simulink model "CMM_iCub_23_25_DoFs"  (Simulink 9.0)
settings: Solver=VariableStepAuto  StartTime=0.0  StopTime=10.0  RelTol=1e-3
libraries: WBToolboxLibrary x31
settings Model: SuppressorTable=22 serialization::archive 11 0 6 0 0 0 1 0  Creator=gnava  LastModifiedBy=gnava
settings DataIOCC: SaveFormat=Dataset
settings OptimizationCC: LifeSpan=auto
settings DebuggingCC: UnderspecifiedInitializationDetection=Simplified  MergeDetectMultiDrivingBlocksExec=error  SFUnexpectedBacktrackingDiag=error  SFNoUnconditionalDefaultTransitionDiag=error  SFExecutionAtInitializationDiag=warning
settings HardwareCC: ProdBitPerPointer=64  ProdBitPerSizeT=64  ProdBitPerPtrDiffT=64  ProdLargestAtomicFloat=Float  ProdIntDivRoundTo=Zero  ProdEndianess=LittleEndian  ProdWordSize=64  ProdHWDeviceType=Intel->x86-64 (Windows64)
settings ModelReferenceCC: PropagateSignalLabelsOutOfModel=on
settings CodeAppCC: StateflowObjectComments=off
settings GRTTargetCC: TargetLangStandard=C99 (ISO)
settings ConfigComp: CovMetricSettings=dwe  CovHtmlReporting=off  CovSaveCumulativeToWorkspaceVar=off  CovSaveSingleToWorkspaceVar=off  CovExternalEMLEnable=on

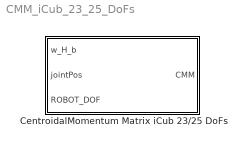
== system CMM_iCub_23_25_DoFs ==
  CentroidalMomentum Matrix iCub 23/25 DoFs : Subsystem

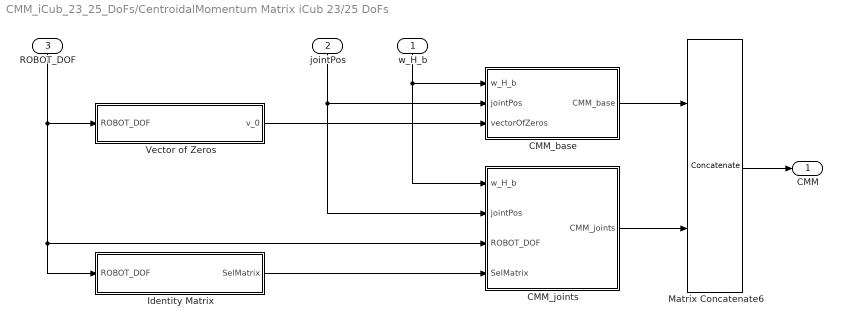
== system CMM_iCub_23_25_DoFs/CentroidalMomentum Matrix iCub 23/25 DoFs ==
  w_H_b : Inport
  jointPos : Inport  Port=2
  ROBOT_DOF : Inport  Port=3
  CMM_base : Subsystem
  CMM_joints : Subsystem
  Identity Matrix : MATLAB Function  TreatAsAtomicUnit=on
  Matrix Concatenate6 : Concatenate  Mode=Multidimensional array  ConcatenateDimension=2
  Vector of Zeros : MATLAB Function  TreatAsAtomicUnit=on
  CMM : Outport
  wires:
  Matrix Concatenate6/1 -> CMM/1
  CMM_base/1(CMM_base) -> Matrix Concatenate6/1
  jointPos/1 -> CMM_joints/2(jointPos), CMM_base/2(jointPos)
  w_H_b/1 -> CMM_joints/1(w_H_b), CMM_base/1(w_H_b)
  ROBOT_DOF/1 -> CMM_joints/3(ROBOT_DOF), Identity Matrix/1(ROBOT_DOF), Vector of Zeros/1(ROBOT_DOF)
  Vector of Zeros/1(v_0) -> CMM_base/3(vectorOfZeros)
  CMM_joints/1(CMM_joints) -> Matrix Concatenate6/2
  Identity Matrix/1(SelMatrix) -> CMM_joints/4(SelMatrix)

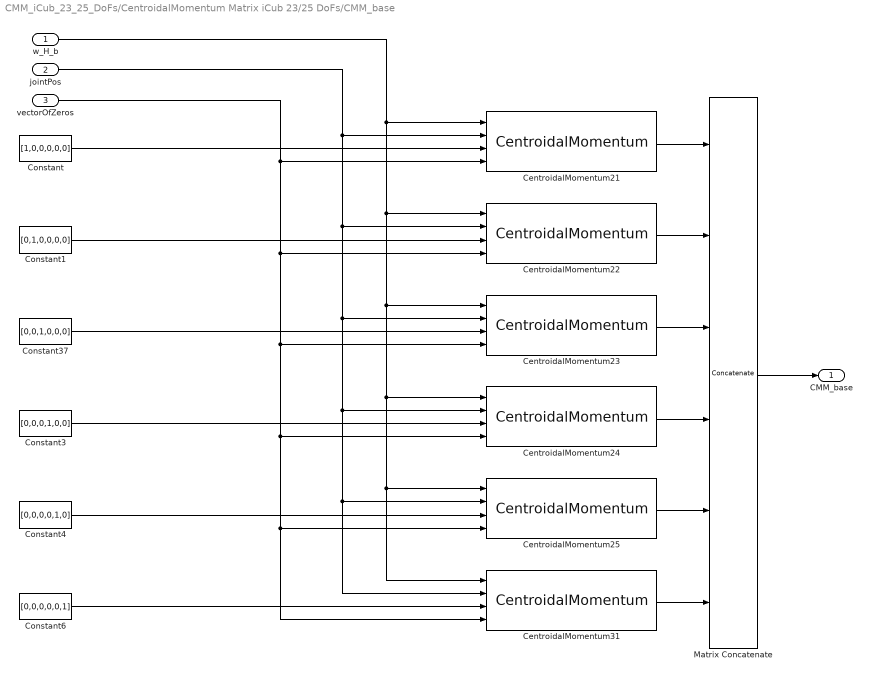
== system CMM_iCub_23_25_DoFs/CentroidalMomentum Matrix iCub 23/25 DoFs/CMM_base ==
  w_H_b : Inport
  jointPos : Inport  Port=2
  vectorOfZeros : Inport  Port=3
  CentroidalMomentum{21..25,31} (6 alike) : WBToolboxLibrary/Model/Dynamics/CentroidalMomentum
      settings: SourceProductName=WholeBodyToolbox
  Constant : Constant  Value=[1,0,0,0,0,0]
  Constant1 : Constant  Value=[0,1,0,0,0,0]
  Constant3 : Constant  Value=[0,0,0,1,0,0]
  Constant37 : Constant  Value=[0,0,1,0,0,0]
  Constant4 : Constant  Value=[0,0,0,0,1,0]
  Constant6 : Constant  Value=[0,0,0,0,0,1]
  Matrix Concatenate : Concatenate  NumInputs=6  Mode=Multidimensional array  ConcatenateDimension=2
  CMM_base : Outport
  wires:
  w_H_b/1 -> CentroidalMomentum31/1, CentroidalMomentum25/1, CentroidalMomentum24/1, CentroidalMomentum23/1, CentroidalMomentum22/1, CentroidalMomentum21/1
  jointPos/1 -> CentroidalMomentum31/2, CentroidalMomentum25/2, CentroidalMomentum24/2, CentroidalMomentum23/2, CentroidalMomentum22/2, CentroidalMomentum21/2
  CentroidalMomentum25/1 -> Matrix Concatenate/5
  Matrix Concatenate/1 -> CMM_base/1
  CentroidalMomentum23/1 -> Matrix Concatenate/3
  CentroidalMomentum24/1 -> Matrix Concatenate/4
  CentroidalMomentum31/1 -> Matrix Concatenate/6
  Constant6/1 -> CentroidalMomentum31/3
  Constant/1 -> CentroidalMomentum21/3
  Constant1/1 -> CentroidalMomentum22/3
  Constant37/1 -> CentroidalMomentum23/3
  vectorOfZeros/1 -> CentroidalMomentum21/4, CentroidalMomentum31/4, CentroidalMomentum25/4, CentroidalMomentum24/4, CentroidalMomentum23/4, CentroidalMomentum22/4
  Constant4/1 -> CentroidalMomentum25/3
  Constant3/1 -> CentroidalMomentum24/3
  CentroidalMomentum22/1 -> Matrix Concatenate/2
  CentroidalMomentum21/1 -> Matrix Concatenate/1

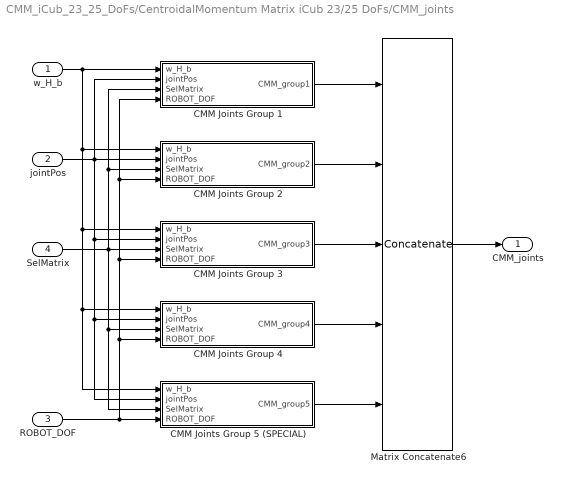
== system CMM_iCub_23_25_DoFs/CentroidalMomentum Matrix iCub 23/25 DoFs/CMM_joints ==
  w_H_b : Inport
  jointPos : Inport  Port=2
  ROBOT_DOF : Inport  Port=3
  SelMatrix : Inport  Port=4
  CMM Joints Group 1 : Subsystem
  CMM Joints Group 2 : Subsystem
  CMM Joints Group 3 : Subsystem
  CMM Joints Group 4 : Subsystem
  CMM Joints Group 5 (SPECIAL) : Subsystem
  Matrix Concatenate6 : Concatenate  NumInputs=5  Mode=Multidimensional array  ConcatenateDimension=2
  CMM_joints : Outport
  wires:
  Matrix Concatenate6/1 -> CMM_joints/1
  w_H_b/1 -> CMM Joints Group 1/1(w_H_b), CMM Joints Group 2/1(w_H_b), CMM Joints Group 3/1(w_H_b), CMM Joints Group 4/1(w_H_b), CMM Joints Group 5 (SPECIAL)/1(w_H_b)
  jointPos/1 -> CMM Joints Group 3/2(jointPos), CMM Joints Group 4/2(jointPos), CMM Joints Group 5 (SPECIAL)/2(jointPos), CMM Joints Group 2/2(jointPos), CMM Joints Group 1/2(jointPos)
  SelMatrix/1 -> CMM Joints Group 4/3(SelMatrix), CMM Joints Group 5 (SPECIAL)/3(SelMatrix), CMM Joints Group 3/3(SelMatrix), CMM Joints Group 2/3(SelMatrix), CMM Joints Group 1/3(SelMatrix)
  CMM Joints Group 1/1(CMM_group1) -> Matrix Concatenate6/1
  CMM Joints Group 2/1(CMM_group2) -> Matrix Concatenate6/2
  CMM Joints Group 3/1(CMM_group3) -> Matrix Concatenate6/3
  CMM Joints Group 4/1(CMM_group4) -> Matrix Concatenate6/4
  CMM Joints Group 5 (SPECIAL)/1(CMM_group5) -> Matrix Concatenate6/5
  ROBOT_DOF/1 -> CMM Joints Group 5 (SPECIAL)/4(ROBOT_DOF), CMM Joints Group 3/4(ROBOT_DOF), CMM Joints Group 1/4(ROBOT_DOF), CMM Joints Group 2/4(ROBOT_DOF), CMM Joints Group 4/4(ROBOT_DOF)

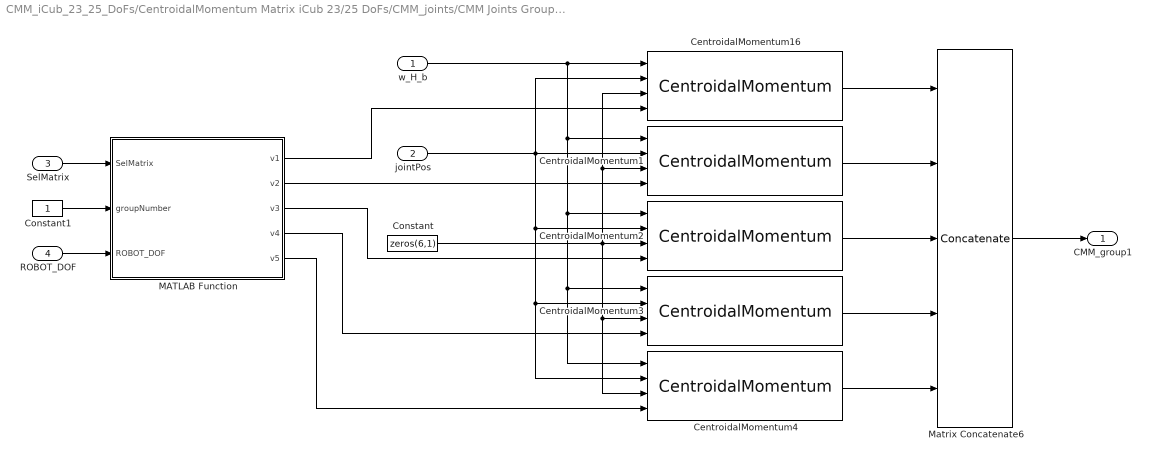
== system CMM_iCub_23_25_DoFs/CentroidalMomentum Matrix iCub 23/25 DoFs/CMM_joints/CMM Joints Group 1 ==
  w_H_b : Inport
  jointPos : Inport  Port=2
  SelMatrix : Inport  Port=3
  ROBOT_DOF : Inport  Port=4
  CentroidalMomentum{1..4,16} (5 alike) : WBToolboxLibrary/Model/Dynamics/CentroidalMomentum
      settings: SourceProductName=WholeBodyToolbox
  Constant : Constant  Value=zeros(6,1)
  Constant1 : Constant
  MATLAB Function : MATLAB Function  TreatAsAtomicUnit=on
  Matrix Concatenate6 : Concatenate  NumInputs=5  Mode=Multidimensional array  ConcatenateDimension=2
  CMM_group1 : Outport
  wires:
  Constant/1 -> CentroidalMomentum4/3, CentroidalMomentum3/3, CentroidalMomentum1/3, CentroidalMomentum16/3, CentroidalMomentum2/3
  CentroidalMomentum2/1 -> Matrix Concatenate6/3
  CentroidalMomentum1/1 -> Matrix Concatenate6/2
  jointPos/1 -> CentroidalMomentum4/2, CentroidalMomentum3/2, CentroidalMomentum2/2, CentroidalMomentum16/2, CentroidalMomentum1/2
  CentroidalMomentum3/1 -> Matrix Concatenate6/4
  CentroidalMomentum16/1 -> Matrix Concatenate6/1
  w_H_b/1 -> CentroidalMomentum1/1, CentroidalMomentum2/1, CentroidalMomentum3/1, CentroidalMomentum4/1, CentroidalMomentum16/1
  CentroidalMomentum4/1 -> Matrix Concatenate6/5
  Matrix Concatenate6/1 -> CMM_group1/1
  MATLAB Function/1(v1) -> CentroidalMomentum16/4
  MATLAB Function/2(v2) -> CentroidalMomentum1/4
  MATLAB Function/3(v3) -> CentroidalMomentum2/4
  MATLAB Function/4(v4) -> CentroidalMomentum3/4
  MATLAB Function/5(v5) -> CentroidalMomentum4/4
  SelMatrix/1 -> MATLAB Function/1(SelMatrix)
  Constant1/1 -> MATLAB Function/2(groupNumber)
  ROBOT_DOF/1 -> MATLAB Function/3(ROBOT_DOF)

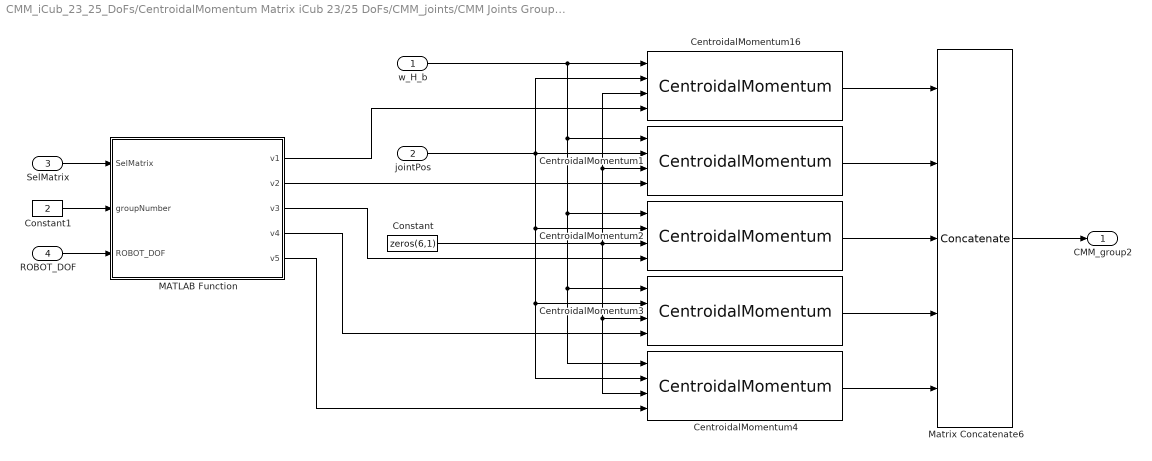
== system CMM_iCub_23_25_DoFs/CentroidalMomentum Matrix iCub 23/25 DoFs/CMM_joints/CMM Joints Group 2 ==
  w_H_b : Inport
  jointPos : Inport  Port=2
  SelMatrix : Inport  Port=3
  ROBOT_DOF : Inport  Port=4
  CentroidalMomentum{1..4,16} (5 alike) : WBToolboxLibrary/Model/Dynamics/CentroidalMomentum
      settings: SourceProductName=WholeBodyToolbox
  Constant : Constant  Value=zeros(6,1)
  Constant1 : Constant  Value=2
  MATLAB Function : MATLAB Function  TreatAsAtomicUnit=on
  Matrix Concatenate6 : Concatenate  NumInputs=5  Mode=Multidimensional array  ConcatenateDimension=2
  CMM_group2 : Outport
  wires:
  Constant/1 -> CentroidalMomentum4/3, CentroidalMomentum3/3, CentroidalMomentum1/3, CentroidalMomentum16/3, CentroidalMomentum2/3
  CentroidalMomentum2/1 -> Matrix Concatenate6/3
  CentroidalMomentum1/1 -> Matrix Concatenate6/2
  jointPos/1 -> CentroidalMomentum4/2, CentroidalMomentum3/2, CentroidalMomentum2/2, CentroidalMomentum16/2, CentroidalMomentum1/2
  CentroidalMomentum3/1 -> Matrix Concatenate6/4
  CentroidalMomentum16/1 -> Matrix Concatenate6/1
  w_H_b/1 -> CentroidalMomentum1/1, CentroidalMomentum2/1, CentroidalMomentum3/1, CentroidalMomentum4/1, CentroidalMomentum16/1
  CentroidalMomentum4/1 -> Matrix Concatenate6/5
  Matrix Concatenate6/1 -> CMM_group2/1
  MATLAB Function/1(v1) -> CentroidalMomentum16/4
  MATLAB Function/2(v2) -> CentroidalMomentum1/4
  MATLAB Function/3(v3) -> CentroidalMomentum2/4
  MATLAB Function/4(v4) -> CentroidalMomentum3/4
  MATLAB Function/5(v5) -> CentroidalMomentum4/4
  SelMatrix/1 -> MATLAB Function/1(SelMatrix)
  Constant1/1 -> MATLAB Function/2(groupNumber)
  ROBOT_DOF/1 -> MATLAB Function/3(ROBOT_DOF)

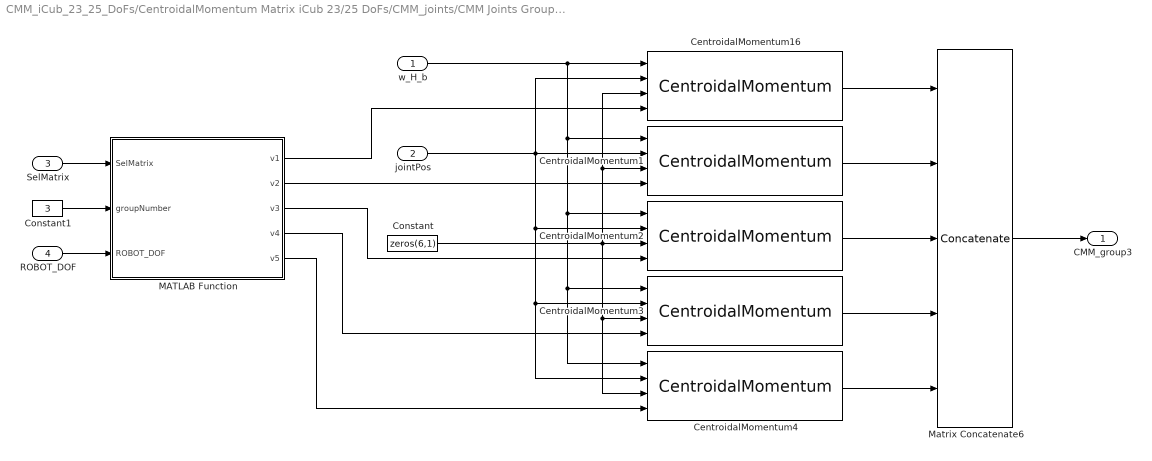
== system CMM_iCub_23_25_DoFs/CentroidalMomentum Matrix iCub 23/25 DoFs/CMM_joints/CMM Joints Group 3 ==
  w_H_b : Inport
  jointPos : Inport  Port=2
  SelMatrix : Inport  Port=3
  ROBOT_DOF : Inport  Port=4
  CentroidalMomentum{1..4,16} (5 alike) : WBToolboxLibrary/Model/Dynamics/CentroidalMomentum
      settings: SourceProductName=WholeBodyToolbox
  Constant : Constant  Value=zeros(6,1)
  Constant1 : Constant  Value=3
  MATLAB Function : MATLAB Function  TreatAsAtomicUnit=on
  Matrix Concatenate6 : Concatenate  NumInputs=5  Mode=Multidimensional array  ConcatenateDimension=2
  CMM_group3 : Outport
  wires:
  Constant/1 -> CentroidalMomentum4/3, CentroidalMomentum3/3, CentroidalMomentum1/3, CentroidalMomentum16/3, CentroidalMomentum2/3
  CentroidalMomentum2/1 -> Matrix Concatenate6/3
  CentroidalMomentum1/1 -> Matrix Concatenate6/2
  jointPos/1 -> CentroidalMomentum4/2, CentroidalMomentum3/2, CentroidalMomentum2/2, CentroidalMomentum16/2, CentroidalMomentum1/2
  CentroidalMomentum3/1 -> Matrix Concatenate6/4
  CentroidalMomentum16/1 -> Matrix Concatenate6/1
  w_H_b/1 -> CentroidalMomentum1/1, CentroidalMomentum2/1, CentroidalMomentum3/1, CentroidalMomentum4/1, CentroidalMomentum16/1
  CentroidalMomentum4/1 -> Matrix Concatenate6/5
  Matrix Concatenate6/1 -> CMM_group3/1
  MATLAB Function/1(v1) -> CentroidalMomentum16/4
  MATLAB Function/2(v2) -> CentroidalMomentum1/4
  MATLAB Function/3(v3) -> CentroidalMomentum2/4
  MATLAB Function/4(v4) -> CentroidalMomentum3/4
  MATLAB Function/5(v5) -> CentroidalMomentum4/4
  SelMatrix/1 -> MATLAB Function/1(SelMatrix)
  Constant1/1 -> MATLAB Function/2(groupNumber)
  ROBOT_DOF/1 -> MATLAB Function/3(ROBOT_DOF)

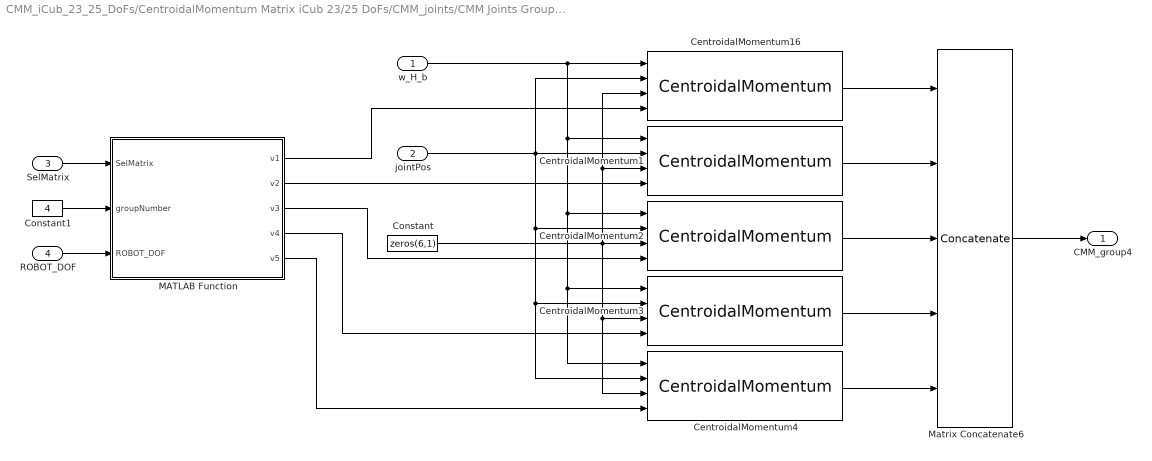
== system CMM_iCub_23_25_DoFs/CentroidalMomentum Matrix iCub 23/25 DoFs/CMM_joints/CMM Joints Group 4 ==
  w_H_b : Inport
  jointPos : Inport  Port=2
  SelMatrix : Inport  Port=3
  ROBOT_DOF : Inport  Port=4
  CentroidalMomentum{1..4,16} (5 alike) : WBToolboxLibrary/Model/Dynamics/CentroidalMomentum
      settings: SourceProductName=WholeBodyToolbox
  Constant : Constant  Value=zeros(6,1)
  Constant1 : Constant  Value=4
  MATLAB Function : MATLAB Function  TreatAsAtomicUnit=on
  Matrix Concatenate6 : Concatenate  NumInputs=5  Mode=Multidimensional array  ConcatenateDimension=2
  CMM_group4 : Outport
  wires:
  Constant/1 -> CentroidalMomentum4/3, CentroidalMomentum3/3, CentroidalMomentum1/3, CentroidalMomentum16/3, CentroidalMomentum2/3
  CentroidalMomentum2/1 -> Matrix Concatenate6/3
  CentroidalMomentum1/1 -> Matrix Concatenate6/2
  jointPos/1 -> CentroidalMomentum4/2, CentroidalMomentum3/2, CentroidalMomentum2/2, CentroidalMomentum16/2, CentroidalMomentum1/2
  CentroidalMomentum3/1 -> Matrix Concatenate6/4
  CentroidalMomentum16/1 -> Matrix Concatenate6/1
  w_H_b/1 -> CentroidalMomentum1/1, CentroidalMomentum2/1, CentroidalMomentum3/1, CentroidalMomentum4/1, CentroidalMomentum16/1
  CentroidalMomentum4/1 -> Matrix Concatenate6/5
  Matrix Concatenate6/1 -> CMM_group4/1
  MATLAB Function/1(v1) -> CentroidalMomentum16/4
  MATLAB Function/2(v2) -> CentroidalMomentum1/4
  MATLAB Function/3(v3) -> CentroidalMomentum2/4
  MATLAB Function/4(v4) -> CentroidalMomentum3/4
  MATLAB Function/5(v5) -> CentroidalMomentum4/4
  SelMatrix/1 -> MATLAB Function/1(SelMatrix)
  Constant1/1 -> MATLAB Function/2(groupNumber)
  ROBOT_DOF/1 -> MATLAB Function/3(ROBOT_DOF)

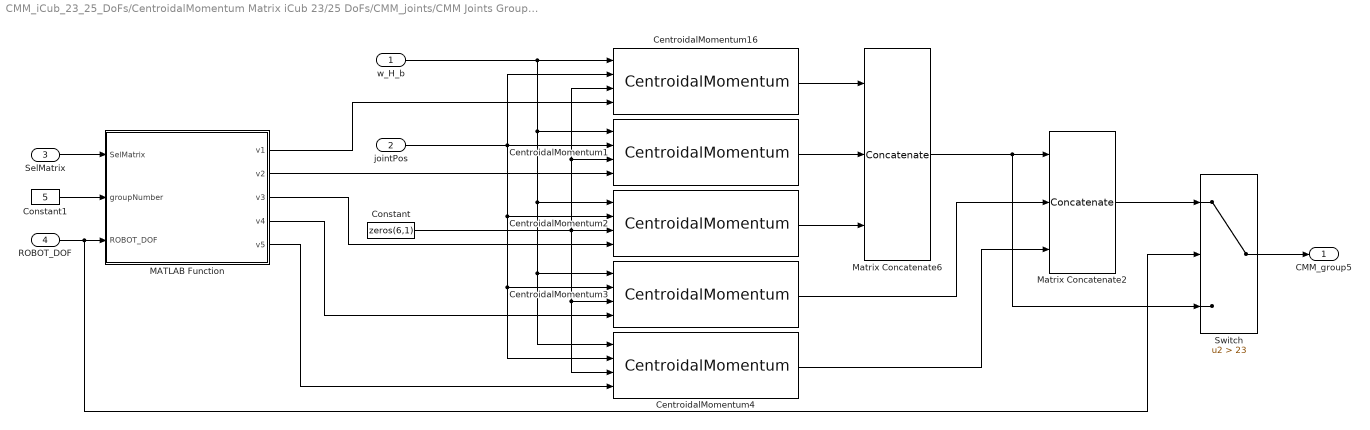
== system CMM_iCub_23_25_DoFs/CentroidalMomentum Matrix iCub 23/25 DoFs/CMM_joints/CMM Joints Group 5 (SPECIAL) ==
  w_H_b : Inport
  jointPos : Inport  Port=2
  SelMatrix : Inport  Port=3
  ROBOT_DOF : Inport  Port=4
  CentroidalMomentum{1..4,16} (5 alike) : WBToolboxLibrary/Model/Dynamics/CentroidalMomentum
      settings: SourceProductName=WholeBodyToolbox
  Constant : Constant  Value=zeros(6,1)
  Constant1 : Constant  Value=5
  MATLAB Function : MATLAB Function  TreatAsAtomicUnit=on
  Matrix Concatenate2 : Concatenate  NumInputs=3  Mode=Multidimensional array  ConcatenateDimension=2
  Matrix Concatenate6 : Concatenate  NumInputs=3  Mode=Multidimensional array  ConcatenateDimension=2
  Switch : Switch  Criteria=u2 > Threshold  Threshold=23
  CMM_group5 : Outport
  wires:
  Constant/1 -> CentroidalMomentum4/3, CentroidalMomentum3/3, CentroidalMomentum1/3, CentroidalMomentum16/3, CentroidalMomentum2/3
  CentroidalMomentum2/1 -> Matrix Concatenate6/3
  CentroidalMomentum1/1 -> Matrix Concatenate6/2
  jointPos/1 -> CentroidalMomentum4/2, CentroidalMomentum3/2, CentroidalMomentum2/2, CentroidalMomentum16/2, CentroidalMomentum1/2
  CentroidalMomentum3/1 -> Matrix Concatenate2/2
  CentroidalMomentum16/1 -> Matrix Concatenate6/1
  w_H_b/1 -> CentroidalMomentum1/1, CentroidalMomentum2/1, CentroidalMomentum3/1, CentroidalMomentum4/1, CentroidalMomentum16/1
  CentroidalMomentum4/1 -> Matrix Concatenate2/3
  MATLAB Function/1(v1) -> CentroidalMomentum16/4
  MATLAB Function/2(v2) -> CentroidalMomentum1/4
  MATLAB Function/3(v3) -> CentroidalMomentum2/4
  MATLAB Function/4(v4) -> CentroidalMomentum3/4
  MATLAB Function/5(v5) -> CentroidalMomentum4/4
  SelMatrix/1 -> MATLAB Function/1(SelMatrix)
  Constant1/1 -> MATLAB Function/2(groupNumber)
  ROBOT_DOF/1 -> Switch/2, MATLAB Function/3(ROBOT_DOF)
  Matrix Concatenate6/1 -> Switch/3, Matrix Concatenate2/1
  Matrix Concatenate2/1 -> Switch/1
  Switch/1 -> CMM_group5/1

== matlab function CentroidalMomentum Matrix iCub 23//25 DoFs/Identity Matrix ==
  data: ROBOT_DOF input double; SelMatrix output double
function SelMatrix = generateSelectorMatrix(ROBOT_DOF)

    if ROBOT_DOF > 23
        
        SelMatrix = eye(ROBOT_DOF);
    else
        SelMatrix = blkdiag(eye(ROBOT_DOF), zeros(2));
    end
end

== matlab function CentroidalMomentum Matrix iCub 23//25 DoFs/Vector of Zeros ==
  data: ROBOT_DOF input double; v_0 output double
function v_0 = generateVectorOfZeros(ROBOT_DOF)

    v_0 = zeros(ROBOT_DOF,1);
end

== matlab function CentroidalMomentum Matrix iCub 23//25 DoFs/CMM_joints/CMM Joints Group 1/MATLAB Function ==
  data: SelMatrix input double; v1 output double; groupNumber input double; v2 output double; v3 output double; v4 output double; v5 output double; ROBOT_DOF input double
function [v1,v2,v3,v4,v5] = selectFiveMatrixColumns(SelMatrix,groupNumber,ROBOT_DOF)

    v1 = SelMatrix((groupNumber-1)*5 + 1,1:ROBOT_DOF);
    v2 = SelMatrix((groupNumber-1)*5 + 2,1:ROBOT_DOF);
    v3 = SelMatrix((groupNumber-1)*5 + 3,1:ROBOT_DOF);
    v4 = SelMatrix((groupNumber-1)*5 + 4,1:ROBOT_DOF);
    v5 = SelMatrix((groupNumber-1)*5 + 5,1:ROBOT_DOF);
end

== matlab function CentroidalMomentum Matrix iCub 23//25 DoFs/CMM_joints/CMM Joints Group 2/MATLAB Function ==
  data: SelMatrix input double; v1 output double; groupNumber input double; v2 output double; v3 output double; v4 output double; v5 output double; ROBOT_DOF input double
function [v1,v2,v3,v4,v5] = selectFiveMatrixColumns(SelMatrix,groupNumber,ROBOT_DOF)

    v1 = SelMatrix((groupNumber-1)*5 + 1,1:ROBOT_DOF);
    v2 = SelMatrix((groupNumber-1)*5 + 2,1:ROBOT_DOF);
    v3 = SelMatrix((groupNumber-1)*5 + 3,1:ROBOT_DOF);
    v4 = SelMatrix((groupNumber-1)*5 + 4,1:ROBOT_DOF);
    v5 = SelMatrix((groupNumber-1)*5 + 5,1:ROBOT_DOF);
end

== matlab function CentroidalMomentum Matrix iCub 23//25 DoFs/CMM_joints/CMM Joints Group 3/MATLAB Function ==
  data: SelMatrix input double; v1 output double; groupNumber input double; v2 output double; v3 output double; v4 output double; v5 output double; ROBOT_DOF input double
function [v1,v2,v3,v4,v5] = selectFiveMatrixColumns(SelMatrix,groupNumber,ROBOT_DOF)

    v1 = SelMatrix((groupNumber-1)*5 + 1,1:ROBOT_DOF);
    v2 = SelMatrix((groupNumber-1)*5 + 2,1:ROBOT_DOF);
    v3 = SelMatrix((groupNumber-1)*5 + 3,1:ROBOT_DOF);
    v4 = SelMatrix((groupNumber-1)*5 + 4,1:ROBOT_DOF);
    v5 = SelMatrix((groupNumber-1)*5 + 5,1:ROBOT_DOF);
end

== matlab function CentroidalMomentum Matrix iCub 23//25 DoFs/CMM_joints/CMM Joints Group 4/MATLAB Function ==
  data: SelMatrix input double; v1 output double; groupNumber input double; v2 output double; v3 output double; v4 output double; v5 output double; ROBOT_DOF input double
function [v1,v2,v3,v4,v5] = selectFiveMatrixColumns(SelMatrix,groupNumber,ROBOT_DOF)

    v1 = SelMatrix((groupNumber-1)*5 + 1,1:ROBOT_DOF);
    v2 = SelMatrix((groupNumber-1)*5 + 2,1:ROBOT_DOF);
    v3 = SelMatrix((groupNumber-1)*5 + 3,1:ROBOT_DOF);
    v4 = SelMatrix((groupNumber-1)*5 + 4,1:ROBOT_DOF);
    v5 = SelMatrix((groupNumber-1)*5 + 5,1:ROBOT_DOF);
end

== matlab function CentroidalMomentum Matrix iCub 23//25 DoFs/CMM_joints/CMM Joints Group 5 (SPECIAL)/MATLAB Function ==
  data: SelMatrix input double; v1 output double; groupNumber input double; v2 output double; v3 output double; v4 output double; v5 output double; ROBOT_DOF input double
function [v1,v2,v3,v4,v5] = selectFiveMatrixColumns(SelMatrix,groupNumber,ROBOT_DOF)

    v1 = SelMatrix((groupNumber-1)*5 + 1,1:ROBOT_DOF);
    v2 = SelMatrix((groupNumber-1)*5 + 2,1:ROBOT_DOF);
    v3 = SelMatrix((groupNumber-1)*5 + 3,1:ROBOT_DOF);
    v4 = SelMatrix((groupNumber-1)*5 + 4,1:ROBOT_DOF);
    v5 = SelMatrix((groupNumber-1)*5 + 5,1:ROBOT_DOF);
end
